simulink model "sparse_encoding_decoding"  (R2021b)
settings: Solver=FixedStepDiscrete  StartTime=0.0  StopTime=1000.0  RelTol=1e-3
libraries: wnnlib x3
settings Model: Creator=20214358  LastModifiedBy=20214358

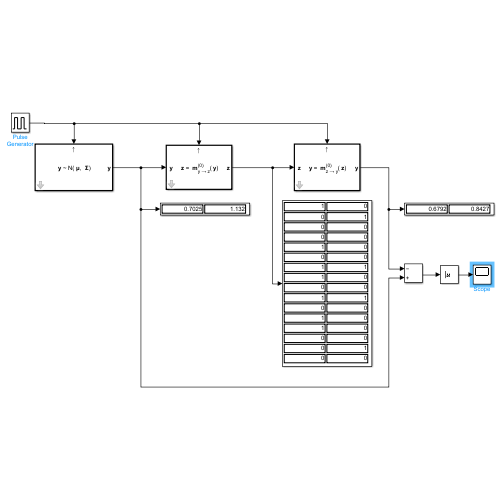
[thumbnail: Simulink's stored preview of the top-level diagram]
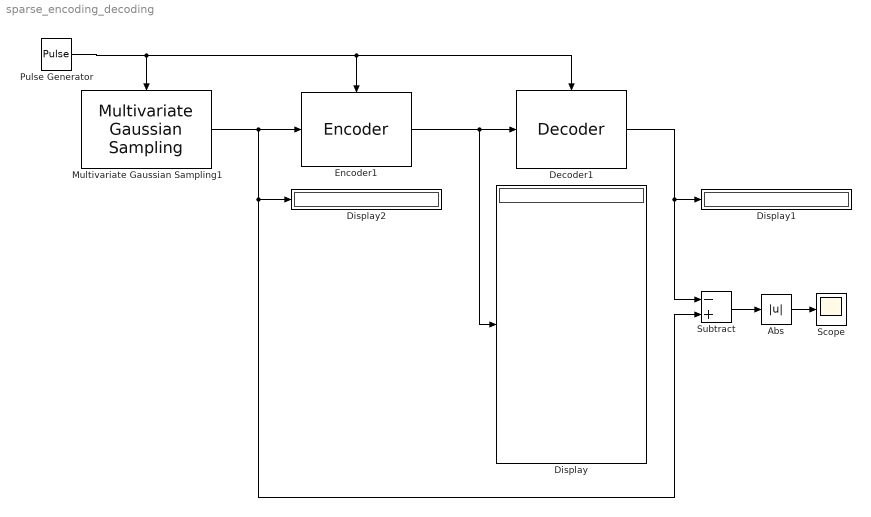
== system sparse_encoding_decoding ==
  Abs : Abs
  Decoder1 : wnnlib/Utilities/Decoder  codec_id=0  output_dims=2  min_bounds=[-10 -10]  max_bounds=[10 10]
      settings: SourceProductName=Weightless Neural Networks Toolbox
  Display : Display
  Display1 : Display
  Display2 : Display
  Encoder1 : wnnlib/Utilities/Encoder  codec_id=0  output_dims=32  learning_rate=0.001  min_splitting_volume=0.001  min_bounds=[-10 -10]  max_bounds=[10 10]
      settings: SourceProductName=Weightless Neural Networks Toolbox
  Multivariate Gaussian Sampling1 : wnnlib/Sources/Multivariate Gaussian Sampling  vecdAvg=[1 1]  matdCov=[2 1; 1 2]  nSeed=0
      settings: SourceProductName=Weightless Neural Networks Toolbox
  Pulse Generator : DiscretePulseGenerator  PulseType=Time based  Period=1  PulseWidth=5
  Scope : Scope
  Subtract : Sum  Inputs=-+
  wires:
  Pulse Generator/1 -> Multivariate Gaussian Sampling1/Trigger, Decoder1/Trigger, Encoder1/Trigger
  Multivariate Gaussian Sampling1/1 -> Encoder1/1, Subtract/2, Display2/1
  Encoder1/1 -> Display/1, Decoder1/1
  Decoder1/1 -> Subtract/1, Display1/1
  Subtract/1 -> Abs/1
  Abs/1 -> Scope/1
